simulink model "zadacha_01"  (Simulink 7.1)
settings: Solver=ode45  StartTime=0.0  StopTime=200  RelTol=1e-3
settings Model: Creator=Slavi  LastModifiedBy=Slavi

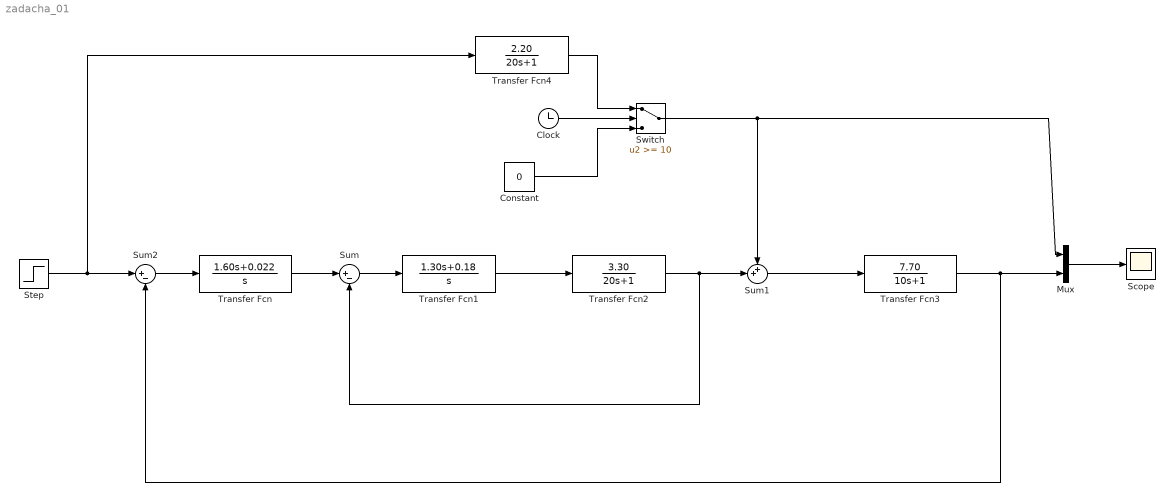
== system zadacha_01 ==
  Clock : Clock
      settings: Decimation=10
  Constant : Constant  Value=0  OutDataType=sfix(16)  OutScaling=2^0
  Mux : Mux  Inputs=2
  Scope : Scope
  Step : Step  Time=0
  Sum : Sum  Inputs=|+-  OutDataType=sfix(16)  OutScaling=2^0
  Sum1 : Sum  Inputs=++|  OutDataType=sfix(16)  OutScaling=2^0
  Sum2 : Sum  Inputs=|+-  OutDataType=sfix(16)  OutScaling=2^0
  Switch : Switch  Threshold=10  OutDataType=sfix(16)  OutScaling=2^0  SaturateOnIntegerOverflow=on  InputSameDT=on
  Transfer Fcn : TransferFcn  Numerator=[1.60 0.022]  Denominator=[1 0]
  Transfer Fcn1 : TransferFcn  Numerator=[1.30 0.18]  Denominator=[1 0]
  Transfer Fcn2 : TransferFcn  Numerator=[3.30]  Denominator=[20 1]
  Transfer Fcn3 : TransferFcn  Numerator=[7.70]  Denominator=[10 1]
  Transfer Fcn4 : TransferFcn  Numerator=[2.20]  Denominator=[20 1]
  wires:
  Transfer Fcn/1 -> Sum/1
  Sum/1 -> Transfer Fcn1/1
  Transfer Fcn1/1 -> Transfer Fcn2/1
  Transfer Fcn2/1 -> Sum1/2, Sum/2
  Sum1/1 -> Transfer Fcn3/1
  Switch/1 -> Sum1/1, Mux/1
  Clock/1 -> Switch/2
  Transfer Fcn4/1 -> Switch/1
  Step/1 -> Transfer Fcn4/1, Sum2/1
  Constant/1 -> Switch/3
  Transfer Fcn3/1 -> Mux/2, Sum2/2
  Mux/1 -> Scope/1
  Sum2/1 -> Transfer Fcn/1
